simulink model "motorWithTF"  (R2021b)
settings: Solver=VariableStepAuto  StartTime=0.0  StopTime=10.0  RelTol=1e-3
values from neighbouring files (symbols this model uses):
  b = 0.5    [Assignment2_Curtis.m]    (also in Assignment2m_Curtis.m)
  J = 0.05    [Assignment2_Curtis.m]    (also in Assignment2m_Curtis.m)
  Ke = 0.5    [Assignment2_Curtis.m]    (also in Assignment2m_Curtis.m)
  Kt = 0.5    [Assignment2_Curtis.m]    (also in Assignment2m_Curtis.m)
  Ra = 1    [Assignment2_Curtis.m]    (also in Assignment2m_Curtis.m)
  velDen = velDen{1}    [Assignment2_Curtis.m]    (also in Assignment2m_Curtis.m)
  velNum = velNum{1}    [Assignment2_Curtis.m]    (also in Assignment2m_Curtis.m)
settings Model: Creator=Alex  LastModifiedBy=Alex

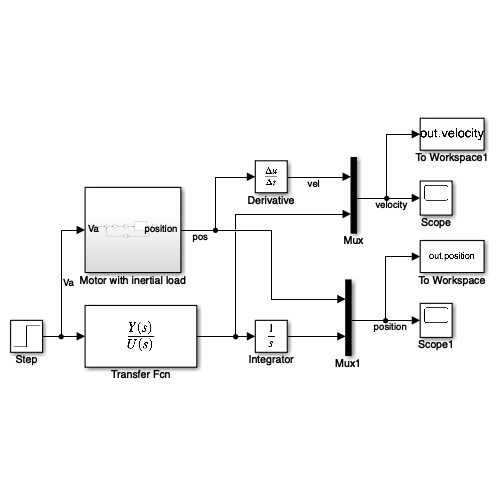
[thumbnail: Simulink's stored preview of the top-level diagram]
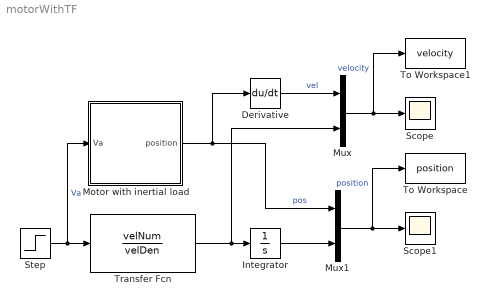
== system motorWithTF ==
  Derivative : Derivative
  Integrator : Integrator
  Motor with inertial load : Subsystem
  Mux : Mux  Inputs=2
  Mux1 : Mux  Inputs=2
  Scope : Scope
  Scope1 : Scope
  Step : Step  SampleTime=0
  To Workspace : ToWorkspace  VariableName=position  SaveFormat=Timeseries  SampleTime=-1
  To Workspace1 : ToWorkspace  VariableName=velocity  SaveFormat=Timeseries  SampleTime=-1
  Transfer Fcn : TransferFcn  Numerator=velNum  Denominator=velDen
  wires:
  Mux/1 -> Scope/1, To Workspace1/1  "velocity"
  Mux1/1 -> Scope1/1, To Workspace/1  "position"
  Transfer Fcn/1 -> Mux/2, Integrator/1
  Step/1 -> Transfer Fcn/1, Motor with inertial load/1(Va)  "Va"
  Derivative/1 -> Mux/1  "vel"
  Motor with inertial load/1(position) -> Mux1/1, Derivative/1  "pos"
  Integrator/1 -> Mux1/2

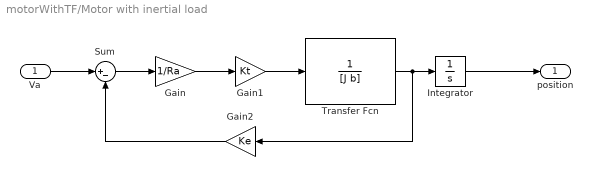
== system motorWithTF/Motor with inertial load ==
  Va : Inport
  Gain : Gain  Gain=1/Ra
  Gain1 : Gain  Gain=Kt
  Gain2 : Gain  Gain=Ke
  Integrator : Integrator
  Sum : Sum  Inputs=|+-
  Transfer Fcn : TransferFcn  Denominator=[J b]
  position : Outport
  wires:
  Va/1 -> Sum/1
  Integrator/1 -> position/1
  Sum/1 -> Gain/1
  Gain/1 -> Gain1/1
  Gain2/1 -> Sum/2
  Transfer Fcn/1 -> Integrator/1, Gain2/1
  Gain1/1 -> Transfer Fcn/1
